simulink model "dc_motor_analogue_pi"  (R2018a)
settings: Solver=VariableStepAuto  StartTime=0.0  StopTime=1000  RelTol=1e-3
undefined symbols (not defined in the file): daq
libraries: daqlib x2
settings Model: Creator=matthew  LastModifiedBy=matthew

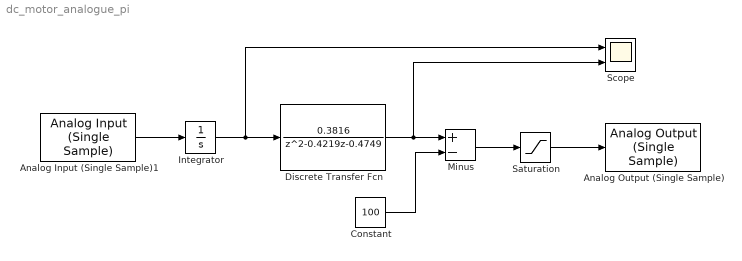
== system dc_motor_analogue_pi ==
  Analog Input (Single Sample)1 : daqlib/Analog Input (Single Sample)  DeviceMenu=ni myDAQ1 (NI myDAQ)  Device=ni myDAQ1 (NI myDAQ)  ObjConstructor=daq.createSession('ni')  BlockSampleTime=1  NChannelsSelected=1  Channels=1$ai0$$myDAQ1$1$2$1$1$#0$ai1$$myDAQ1$1$2$1$1$#  NPorts=1 for all channels  OutputTimestamp=off
      settings: SourceProductName=Data Acquisition Toolbox  SourceProductBaseCode=DA
  Analog Output (Single Sample) : daqlib/Analog Output (Single Sample)  DeviceMenu=ni myDAQ1 (NI myDAQ)  Device=ni myDAQ1 (NI myDAQ)  ObjConstructor=daq.createSession('ni')  NChannelsSelected=1  Channels=1$ao0$$myDAQ1$1$2$N/A$#0$ao1$$myDAQ1$1$2$N/A$#  NPorts=1 for all channels  BlockSampleTime=1
      settings: SourceProductName=Data Acquisition Toolbox  SourceProductBaseCode=DA
  Constant : Constant  Value=100
  Discrete Transfer Fcn : DiscreteTransferFcn  Numerator=[0.3816]  Denominator=[1 -0.4219 -0.4749]
  Integrator : Integrator  LimitOutput=on  UpperSaturationLimit=64  LowerSaturationLimit=-64
  Minus : Sum  Inputs=+-
  Saturation : Saturate  UpperLimit=10  LowerLimit=-10
  Scope : Scope  NumInputPorts=2
  wires:
  Discrete Transfer Fcn/1 -> Scope/2, Minus/1
  Constant/1 -> Minus/2
  Minus/1 -> Saturation/1
  Saturation/1 -> Analog Output (Single Sample)/1
  Integrator/1 -> Scope/1, Discrete Transfer Fcn/1
  Analog Input (Single Sample)1/1 -> Integrator/1
